simulink model "hybrid1"  (Simulink 8.5)
settings: Solver=ode4  SolverMode=SingleTasking  StartTime=0  StopTime=1369  FixedStep=0.0005  RelTol=1e-3
PreLoadFcn:
  | cd Extensions/Simulink/hybrid1
  | hybrid1_sim_init
  | cd ../../..
undefined symbols (not defined in the file or in its folder): enable_stop, eng_consum_fuel, eng_ctrl_max_trq, eng_idle_spd, eng_map_trq, eng_pwr_max, eng_pwr_opt, eng_spd_opt, ess_cap_scale, ess_fixtemp, ess_init_soc, ess_max_ah_cap, ess_max_volts, ess_min_volts, ess_module_num, ess_res_scale_coef, ess_res_scale_fun, ess_tmp, FR, g_eff_map, g_max_spd, g_max_trq, gc_ki_on, gc_kp_on, I_e, I_g, I_m, I_r, I_R2, m_eff_map, m_map_spd, m_max_trq, m_min_volts, max_gen_spd, min_gen_spd, P_eng_mode, P_ev_mode, regstop_soc, soc_control, target_soc, time_step, tx_pg_r, tx_pg_s, w_engine_on
undefined symbols (not defined in the file): ess_r_chg, ess_r_dis, ess_soc, ess_voc
libraries: Solver_SF x1
(part 1 of 2)
settings Model: Creator=hueipeng  LastModifiedBy=ywata  ExtModeTrigMode=oneshot  ExtModeArmWhenConnect=off
settings DataIOCC: LimitDataPoints=off  SaveOutput=off  SaveTime=off  SignalLoggingName=sigsOut
settings OptimizationCC: BooleanDataType=off  OptimizeBlockIOStorage=off  BufferReuse=off  GlobalBufferReuse=off  ExpressionFolding=off  ExpressionDepthLimit=128  LocalBlockOutputs=off  InitFltsAndDblsToZero=on
settings DebuggingCC: SaveWithParameterizedLinksMsg=none  SignalResolutionControl=TryResolveAllWithWarning  MultiTaskDSMMsg=warning  MultiTaskCondExecSysMsg=none  FcnCallInpInsideContextMsg=EnableAllAsError
settings HardwareCC: TargetUnknown=on
settings GRTTargetCC: TargetFcnLib=ansi_tfl_tmw.mat

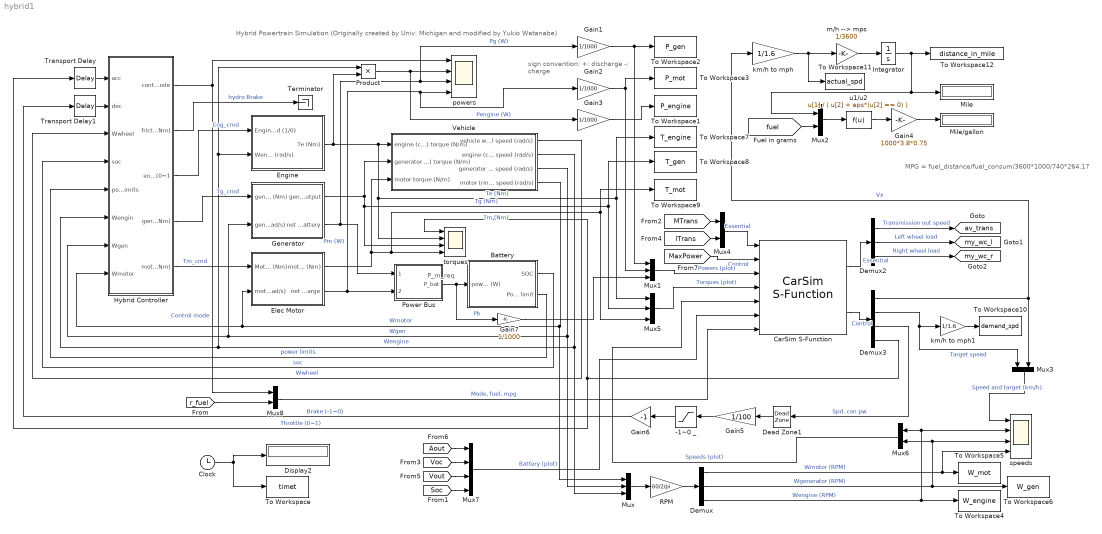
== system hybrid1 ==
  note: Hybrid Powertrain Simulation (Originally created by Univ. Michigan and modified by Yukio Watanabe)
  note: P_m_req
  note: sign convention:
      | +: discharge     -: charge
  note: MPG = fuel_distance/fuel_consum/3600*1000/740*264.17
  -1~0 _ : Saturate  UpperLimit=0  LowerLimit=-1
  Battery : Subsystem
      mask Display: disp('Battery')
  CarSim S-Function : Solver_SF/CarSim S-Function  Priority=1  SIMFILE=simfile.sim
  Clock : Clock
  Dead Zone1 : DeadZone  UpperValue=0  SaturateOnIntegerOverflow=on
  Demux : Demux  Outputs=3
  Demux2 : Demux  Outputs=3
  Demux3 : Demux
  Display2 : Display
  Elec Motor : Subsystem
      mask Display: disp('Electric\nMotor')
  Engine : Subsystem
      mask Display: disp('Engine')
  Gain{1..3,7} (4 alike) : Gain  Gain=1/1000  SaturateOnIntegerOverflow=on  OutDataTypeStr=Inherit: Same as input  ParamDataTypeStr=Inherit: Same as input
  Gain4 : Gain  Gain=1000*3.8*0.75  SaturateOnIntegerOverflow=on  OutDataTypeStr=Inherit: Same as input  ParamDataTypeStr=Inherit: Same as input
  Gain5 : Gain  Gain=1/100  SaturateOnIntegerOverflow=on  OutDataTypeStr=Inherit: Same as input  ParamDataTypeStr=Inherit: Same as input
  Gain6 : Gain  Gain=-1  SaturateOnIntegerOverflow=on  OutDataTypeStr=Inherit: Same as input  ParamDataTypeStr=Inherit: Same as input
  Generator : Subsystem
      mask Display: disp('Generator')
  Hybrid Controller : Subsystem
      mask Display: disp('Hybrid\nController')
  Integrator : Integrator  LowerSaturationLimit=0
  Mile : Display
  Mile/gallon : Display
  Mux : Mux  Inputs=3
  Mux1 : Mux  Inputs=3
  Mux{2..4,6,8} (5 alike) : Mux  Inputs=2
  Mux5 : Mux  Inputs=3
  Mux7 : Mux
  Power Bus : Subsystem
      mask Display: disp('Power\nBus')
  Product : Product  SaturateOnIntegerOverflow=on  OutDataTypeStr=Inherit: Same as first input
  RPM : Gain  Gain=60/2/pi  SaturateOnIntegerOverflow=on  OutDataTypeStr=Inherit: Same as input  ParamDataTypeStr=Inherit: Same as input
  Terminator : Terminator
  To Workspace : ToWorkspace  VariableName=timet  SampleTime=time_step
  To Workspace1 : ToWorkspace  VariableName=P_engine  SampleTime=time_step
  To Workspace10 : ToWorkspace  VariableName=demand_spd  SampleTime=time_step
  To Workspace11 : ToWorkspace  VariableName=actual_spd  SampleTime=time_step
  To Workspace12 : ToWorkspace  VariableName=distance_in_mile  SampleTime=time_step
  To Workspace2 : ToWorkspace  VariableName=P_gen  SampleTime=time_step
  To Workspace3 : ToWorkspace  VariableName=P_mot  SampleTime=time_step
  To Workspace4 : ToWorkspace  VariableName=W_engine  SampleTime=time_step
  To Workspace5 : ToWorkspace  VariableName=W_mot  SampleTime=time_step
  To Workspace6 : ToWorkspace  VariableName=W_gen  SampleTime=time_step
  To Workspace7 : ToWorkspace  VariableName=T_engine  SampleTime=time_step
  To Workspace8 : ToWorkspace  VariableName=T_gen  SampleTime=time_step
  To Workspace9 : ToWorkspace  VariableName=T_mot  SampleTime=time_step
  Transport Delay : TransportDelay  DelayTime=0
  Transport Delay1 : TransportDelay  DelayTime=0
  Vehicle : Subsystem
      mask Display: disp('Planetary Gear Set')
  km/h to mph : Gain  Gain=1/1.6  SaturateOnIntegerOverflow=on  OutDataTypeStr=Inherit: Same as input  ParamDataTypeStr=Inherit: Same as input
  km/h to mph1 : Gain  Gain=1/1.6  SaturateOnIntegerOverflow=on  OutDataTypeStr=Inherit: Same as input  ParamDataTypeStr=Inherit: Same as input
  m/h --> mps : Gain  Gain=1/3600  SaturateOnIntegerOverflow=on  OutDataTypeStr=Inherit: Same as input  ParamDataTypeStr=Inherit: Same as input
  powers : Scope  NumInputPorts=4
      settings: TimeRange=29.9995  YMin=0~0~-20000~-20000  YMax=3~40000~30000~40000  SaveName=ScopeData15
  speeds : Scope  NumInputPorts=4
      settings: TickLabels=on  TimeRange=30  YMin=0~0~-5000~0  YMax=100~4000~10000~6000  SaveName=ScopeData8
  torques : Scope  NumInputPorts=4
      settings: TickLabels=on  TimeRange=29.9995  YMin=0~0~-100~-100  YMax=1~100~50~300  SaveName=ScopeData7
  u1/u2 : Fcn  Expr=u[1] / ( u[2] + eps*(u[2] == 0) )
  tag scope: av_trans=global, my_wc_l=global, my_wc_r=global
  wires:
  Power Bus/1(P_bat) -> Gain7/1, Battery/1(power req'd into bus (W))  "Pb"
  Battery/1(SOC) -> Hybrid Controller/4(soc)  "soc"
  Hybrid Controller/3(engine command (0~1) -> Engine/1(Engine on/off cmd (1/0))  "Eng_cmd"
  Hybrid Controller/4(generator torque command (Nm)) -> Generator/1(generator command Torque (Nm))  "Tg_cmd"
  Hybrid Controller/5(motor torque command (Nm)) -> Elec Motor/1(Motor demand Torque (Nm))  "Tm_cmd"
  Elec Motor/2(net Power >0 discharge  <0 charge) -> Power Bus/2(P_motor), powers/4, Gain2/1  "Pm (W)"
  Generator/2(net Power <0 charge the battery  >0 discharge the battery) -> Power Bus/1(P_generator), powers/3, Gain1/1  "Pg (W)"
  Hybrid Controller/2(friction brake torque (Nm)) -> Terminator/1  "hydro Brake"
  Engine/1(Te (Nm)) -> torques/2, Mux5/1, To Workspace7/1, Vehicle/1(engine (carrier) torque (N/m)), Product/2  "Te (Nm)"
  Vehicle/1(vehicle wheel speed (rad/s)) -> Hybrid Controller/3(Wwheel)  "Wwheel"
  Vehicle/2(engine (carrier) speed (rad/s)) -> Hybrid Controller/6(Wengin), Engine/2(Wengine (rad/s)), Product/1, Mux/3  "Wengine"
  Vehicle/3(generator (sun gear) speed (rad/s)) -> Hybrid Controller/7(Wgen), Generator/2(generator speed (rad/s)), Mux/2  "Wgen"
  Vehicle/4(motor (ring gear) speed (rad/s)) -> Mux/1, Hybrid Controller/8(Wmotor), Elec Motor/2(motor speed (rad/s))  "Wmotor"
  Generator/1(generator torque output) -> torques/3, Mux5/2, To Workspace8/1, Vehicle/2(generator (sun gear) torque (N/m))  "Tg (Nm)"
  Elec Motor/1(motor torque output (Nm)) -> Vehicle/3(motor torque (N/m)), Mux5/3, To Workspace9/1, torques/4  "Tm (Nm)"
  Battery/2(Power limit) -> Hybrid Controller/5(power limits)  "power limits"
  Product/1 -> powers/2, Gain3/1  "Pengine (W)"
  RPM/1 -> Demux/1
  Mux/1 -> RPM/1
  Demux/1 -> speeds/4, To Workspace5/1  "Wmotor (RPM)"
  Demux/2 -> speeds/3, Mux6/2, To Workspace6/1  "Wgenerator (RPM)"
  Demux/3 -> speeds/2, Mux6/1, To Workspace4/1  "Wengine (RPM)"
  Clock/1 -> Display2/1, To Workspace/1
  Gain1/1 -> Mux1/1, To Workspace2/1
  Gain2/1 -> To Workspace3/1, Mux1/2
  Gain3/1 -> To Workspace1/1
  Integrator/1 -> Mux2/1, Mile/1, To Workspace12/1
  [fuel] -> Mux2/2
  u1/u2/1 -> Gain4/1
  Gain4/1 -> Mile/gallon/1
  Mux2/1 -> u1/u2/1
  [MTrans] -> Mux4/1
  Demux2/1 -> [av_trans]  "Transmission out speed"
  Demux2/2 -> [my_wc_l]  "Left wheel load"
  Demux2/3 -> [my_wc_r]  "Right wheel load"
  Demux3/1 -> km/h to mph/1, Mux3/2  "Vx"
  Demux3/4 -> torques/1, Transport Delay/1  "Throttle (0~1)"
  Demux3/2 -> Mux3/1, km/h to mph1/1  "Target speed"
  [ITrans] -> Mux4/2
  [MaxPower] -> CarSim S-Function/2  "Control"
  km/h to mph1/1 -> To Workspace10/1
  Demux3/3 -> Dead Zone1/1  "Spd. con pw"
  Dead Zone1/1 -> Gain5/1
  Gain5/1 -> -1~0 _/1
  -1~0 _/1 -> Gain6/1
  Gain6/1 -> Transport Delay1/1  "Brake (-1~0)"
  m/h --> mps/1 -> Integrator/1
  km/h to mph/1 -> To Workspace11/1, m/h --> mps/1
  Mux3/1 -> speeds/1  "Speed and target (km/h)"
  Transport Delay/1 -> Hybrid Controller/1(acc)
  Transport Delay1/1 -> Hybrid Controller/2(dec)
  Hybrid Controller/1(control mode) -> Mux8/1, powers/1  "Control mode"
  Mux4/1 -> CarSim S-Function/1  "Essential"
  Mux5/1 -> CarSim S-Function/4  "Torques (plot)"
  Mux6/1 -> CarSim S-Function/5  "Speeds (plot)"
  CarSim S-Function/1 -> Demux2/1  "Essential"
  CarSim S-Function/2 -> Demux3/1  "Control"
  Mux1/1 -> CarSim S-Function/3  "Powers (plot)"
  Gain7/1 -> Mux1/3
  [Aout] -> Mux7/1
  [Voc] -> Mux7/2
  [Vout] -> Mux7/3
  [Soc] -> Mux7/4
  Mux7/1 -> CarSim S-Function/6  "Battery (plot)"
  [r_fuel] -> Mux8/2
  Mux8/1 -> CarSim S-Function/7  "Mode, fuel, mpg"

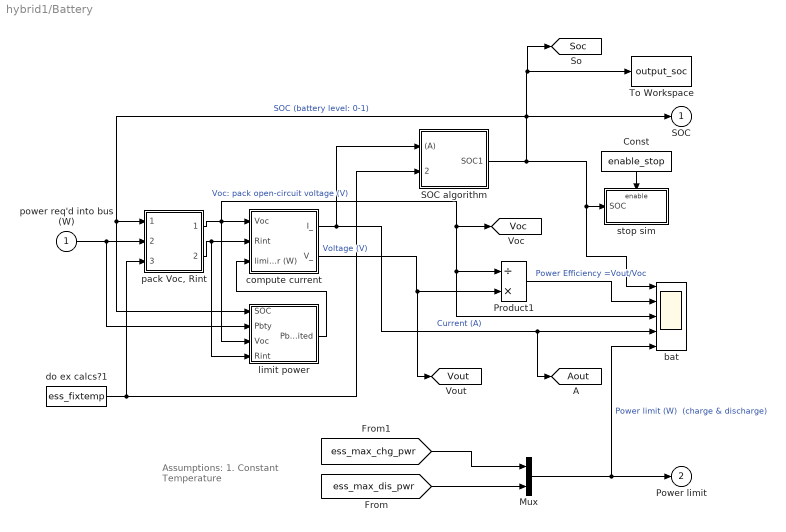
== system hybrid1/Battery ==
  note: Assumptions:
      | 1. Constant Temperature
  power req'd into bus (W) : Inport
  Const : Constant  Value=enable_stop
  Mux : Mux  Inputs=2
  Product1 : Product  Inputs=/*  SaturateOnIntegerOverflow=on  InputSameDT=on  OutDataTypeStr=Inherit: Same as first input
  SOC algorithm : Subsystem  AncestorBlock=|
      | lib_energy_storage/Ess Choices/energy
      | storage <ess>/SOC
      | algorithm
      mask Display: disp('SOC\nalgorithm')
  To Workspace : ToWorkspace  VariableName=output_soc  SampleTime=time_step
  bat : Scope  NumInputPorts=5
      settings: TimeRange=30  YMin=0.5300000000000001~0.6000000000000001~308.8~-50~-50000  YMax=0.6200000000000001~1.2~309.2~100~50000
  compute current : Subsystem  AncestorBlock=|
      | lib_energy_storage/Ess Choices/energy
      | storage <ess>/compute
      | current
      mask Display: disp('Compute\nCurrent')
  do ex calcs?1 : Constant  Value=ess_fixtemp
  limit power : Subsystem  AncestorBlock=lib_energy_storage/Ess Choices/energy storage <ess>/limit power
      mask Display: disp('Limit\nPower')
  "pack Voc, Rint" : Subsystem  AncestorBlock=|
      | lib_energy_storage/Ess Choices/energy
      | storage <ess>/pack
      | Voc, Rint
      mask Display: disp('Pack\nVoc,Rint')
  stop sim : Subsystem  AncestorBlock=lib_energy_storage/Ess Choices/energy storage <ess>/stop sim  TreatAsAtomicUnit=on
  SOC : Outport  InitialOutput=0
  Power limit : Outport  Port=2  InitialOutput=0
  tag scope: Aout=global, Soc=global, Voc=global, Vout=global
  wires:
  limit power/1("Pbty, limited") -> compute current/3(limited output power (W))
  "pack Voc, Rint"/1(pack open- circuit voltage) -> limit power/3(Voc), compute current/1(Voc), Product1/1, bat/3, [Voc]  "Voc: pack open-circuit voltage (V)"
  "pack Voc, Rint"/2(pack resistance) -> compute current/2(Rint), limit power/4(Rint)
  Const/1 -> stop sim/Enable
  SOC algorithm/1(SOC1) -> limit power/1(SOC), "pack Voc, Rint"/1(SOC (prev)), SOC/1, [Soc], To Workspace/1, bat/1, stop sim/1(SOC)  "SOC (battery level: 0-1)"
  compute current/1(I_) -> SOC algorithm/1((A)), [Aout], bat/4  "Current (A)"
  power req'd into bus (W)/1 -> "pack Voc, Rint"/2(req'd battery power (W)), limit power/2(Pbty)
  compute current/2(V_) -> [Vout], Product1/2  "Voltage (V)"
  do ex calcs?1/1 -> "pack Voc, Rint"/3(mod tmp   (C)), SOC algorithm/2(tmp (C))
  Mux/1 -> Power limit/1, bat/5  "Power limit (W)  (charge & discharge)"
  Product1/1 -> bat/2  "Power Efficiency =Vout/Voc"
  [ess_max_dis_pwr] -> Mux/2
  [ess_max_chg_pwr] -> Mux/1

== system hybrid1/Elec Motor ==
  note: disch
  note: charge
  note: discharging
      | power
  Motor demand Torque (Nm) : Inport
  motor speed (rad/s) : Inport  Port=2
  Abs : Abs  SaturateOnIntegerOverflow=on
  Efficiency Look-Up Table (2-D) : Lookup2D  RowIndex=m_map_spd  ColumnIndex=m_map_trq  Table=m_eff_map  SaturateOnIntegerOverflow=on  InputSameDT=on
  First-order lag : TransferFcn  Denominator=[0.05 1]
  MinMax : MinMax  Inputs=2  SaturateOnIntegerOverflow=on  InputSameDT=on
  Power out  is > 0 or < 0 ? : Switch  SaturateOnIntegerOverflow=on  InputSameDT=on
  Product1 : Product  Inputs=*/  SaturateOnIntegerOverflow=on  InputSameDT=on  OutDataTypeStr=Inherit: Same as first input
  Sign : Signum
  charging power : Product  SaturateOnIntegerOverflow=on  InputSameDT=on  OutDataTypeStr=Inherit: Same as first input
  max torque : Lookup  InputValues=m_map_spd  Table=m_max_trq  SaturateOnIntegerOverflow=on
  motoring or braking torque2 : Product  SaturateOnIntegerOverflow=on  InputSameDT=on  OutDataTypeStr=Inherit: Same as first input
  power1 : Product  SaturateOnIntegerOverflow=on  InputSameDT=on  OutDataTypeStr=Inherit: Same as first input
  motor torque output (Nm) : Outport  InitialOutput=0
  net Power >0 discharge  <0 charge : Outport  Port=2  InitialOutput=0
  wires:
  charging power/1 -> Power out  is > 0 or < 0 ?/3
  Product1/1 -> Power out  is > 0 or < 0 ?/1
  Power out  is > 0 or < 0 ?/1 -> net Power >0 discharge  <0 charge/1  "power to/from battery (W)"
  motor speed (rad/s)/1 -> Efficiency Look-Up Table (2-D)/1, motoring or braking torque2/1, max torque/1  "motor speed"
  Motor demand Torque (Nm)/1 -> Abs/1, Sign/1
  power1/1 -> First-order lag/1  "torque"
  Efficiency Look-Up Table (2-D)/1 -> Product1/2, charging power/2
  motoring or braking torque2/1 -> Product1/1, charging power/1, Power out  is > 0 or < 0 ?/2
  Abs/1 -> MinMax/2
  max torque/1 -> MinMax/1
  MinMax/1 -> power1/1
  Sign/1 -> power1/2
  First-order lag/1 -> Efficiency Look-Up Table (2-D)/2, motoring or braking torque2/2, motor torque output (Nm)/1

== system hybrid1/Engine ==
  note: MPG = fuel_distance/fuel_consum/3600*1000/740*264.17
  Engine on/off cmd (1/0) : Inport
  Wengine (rad/s) : Inport  Port=2
  Gain : Gain  Gain=1/1000
  Integrator : Integrator  UpperSaturationLimit=20.5  LowerSaturationLimit=0
  Scope : Scope
      settings: SaveName=ScopeData13
  To Workspace : ToWorkspace  VariableName=fuel_consum_in_g  SampleTime=time_step
  "We, Te to fuel" : Lookup2D  RowIndex=eng_consum_spd  ColumnIndex=eng_consum_trq  Table=eng_consum_fuel  SaturateOnIntegerOverflow=on  InputSameDT=on
  "fuel, speed to T" : Lookup2D  RowIndex=eng_map_spd  ColumnIndex=eng_map_fuel  Table=eng_map_trq  SaturateOnIntegerOverflow=on  InputSameDT=on
  Te (Nm) : Outport
  tag scope: fuel=global, r_fuel=global
  wires:
  Engine on/off cmd (1/0)/1 -> Scope/1, "fuel, speed to T"/2
  Wengine (rad/s)/1 -> "fuel, speed to T"/1, "We, Te to fuel"/1
  "fuel, speed to T"/1 -> Te (Nm)/1, "We, Te to fuel"/2
  "We, Te to fuel"/1 -> Gain/1, Integrator/1
  Integrator/1 -> To Workspace/1, [fuel]
  Gain/1 -> [r_fuel]

== system hybrid1/Generator ==
  note: disch
  note: charge
  note: discharging
      | power
  generator command Torque (Nm) : Inport
  generator speed (rad/s) : Inport  Port=2
  Abs : Abs  SaturateOnIntegerOverflow=on
  Efficiency Look-Up Table (2-D) : Lookup2D  RowIndex=g_map_spd  ColumnIndex=g_map_trq  Table=g_eff_map  SaturateOnIntegerOverflow=on  InputSameDT=on
  First-order lag : TransferFcn  Denominator=[0.05 1]
  MinMax : MinMax  Inputs=2  SaturateOnIntegerOverflow=on  InputSameDT=on
  Power out  is > 0 or < 0 ? : Switch  SaturateOnIntegerOverflow=on  InputSameDT=on
  Product1 : Product  Inputs=*/  SaturateOnIntegerOverflow=on  InputSameDT=on  OutDataTypeStr=Inherit: Same as first input
  Sign : Signum
  charging power : Product  SaturateOnIntegerOverflow=on  InputSameDT=on  OutDataTypeStr=Inherit: Same as first input
  max torque : Lookup  InputValues=g_max_spd  Table=g_max_trq  SaturateOnIntegerOverflow=on
  motoring or braking torque2 : Product  SaturateOnIntegerOverflow=on  InputSameDT=on  OutDataTypeStr=Inherit: Same as first input
  power1 : Product  SaturateOnIntegerOverflow=on  InputSameDT=on  OutDataTypeStr=Inherit: Same as first input
  generator torque output : Outport  InitialOutput=0
  net Power <0 charge the battery  >0 discharge the battery : Outport  Port=2  InitialOutput=0
  wires:
  charging power/1 -> Power out  is > 0 or < 0 ?/3
  Product1/1 -> Power out  is > 0 or < 0 ?/1
  Power out  is > 0 or < 0 ?/1 -> net Power <0 charge the battery  >0 discharge the battery/1  "power to/from battery (W)"
  generator speed (rad/s)/1 -> Efficiency Look-Up Table (2-D)/1, motoring or braking torque2/1, max torque/1  "generator speed"
  generator command Torque (Nm)/1 -> Abs/1, Sign/1
  power1/1 -> First-order lag/1  "torque"
  Efficiency Look-Up Table (2-D)/1 -> Product1/2, charging power/2
  motoring or braking torque2/1 -> Product1/1, charging power/1, Power out  is > 0 or < 0 ?/2
  Abs/1 -> MinMax/2
  max torque/1 -> MinMax/1
  MinMax/1 -> power1/1
  Sign/1 -> power1/2
  First-order lag/1 -> generator torque output/1, Efficiency Look-Up Table (2-D)/2, motoring or braking torque2/2

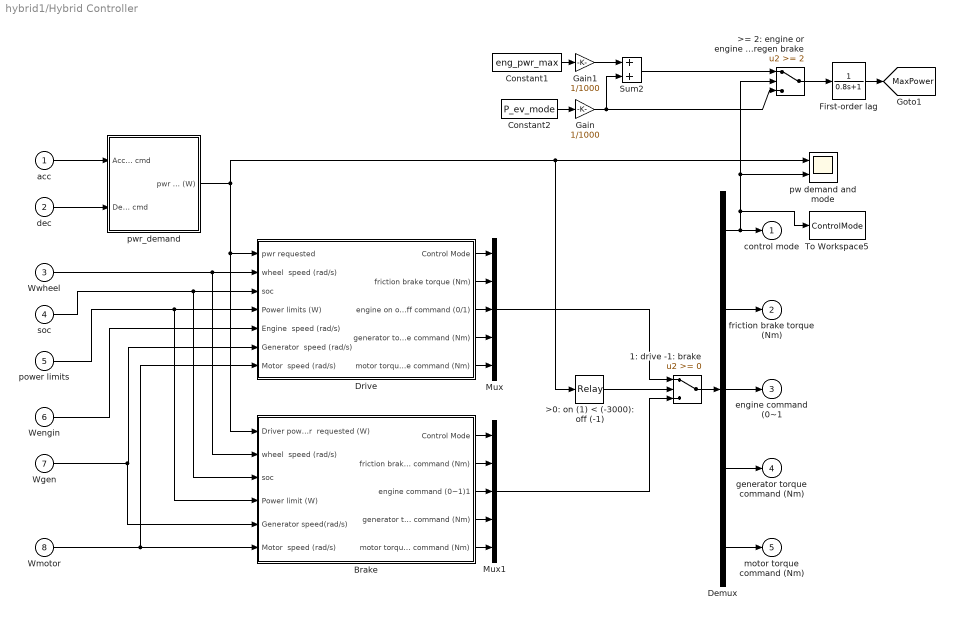
== system hybrid1/Hybrid Controller ==
  acc : Inport
  dec : Inport  Port=2
  Wwheel : Inport  Port=3
  soc : Inport  Port=4
  power limits : Inport  Port=5
  Wengin : Inport  Port=6
  Wgen : Inport  Port=7
  Wmotor : Inport  Port=8
  1: drive -1: brake : Switch  SaturateOnIntegerOverflow=on
  >0: on (1) < (-3000): off (-1) : Relay  OnSwitchValue=0  OffSwitchValue=-3000  OffOutputValue=-1
  >= 2: engine or engine + motor; < 2: motor only or regen brake : Switch  Threshold=2  SaturateOnIntegerOverflow=on
  Brake : Subsystem  AncestorBlock=|
      | lib_controls/<vc> prius/Coordinated
      |  Controller/max engine
      | efficiency point
      mask Display: disp('Braking\nControl')
  Constant1 : Constant  Value=eng_pwr_max
  Constant2 : Constant  Value=P_ev_mode
  Demux : Demux  Outputs=5
  Drive : Subsystem  AncestorBlock=|
      | lib_controls/<vc> prius/Coordinated
      |  Controller/max engine
      | efficiency point
      mask Display: disp('Driving\nControl')
  First-order lag : TransferFcn  Denominator=[0.8 1]
  Gain : Gain  Gain=1/1000
  Gain1 : Gain  Gain=1/1000
  Mux : Mux  Inputs=5
  Mux1 : Mux  Inputs=5
  Sum2 : Sum  SaturateOnIntegerOverflow=on  InputSameDT=on  OutDataTypeStr=Inherit: Same as first input
  To Workspace5 : ToWorkspace  VariableName=ControlMode  SampleTime=time_step
  pw demand and mode : Scope  NumInputPorts=2
      settings: TimeRange=30  YMin=-10000~0  YMax=60000~3  SaveName=ScopeData17
  pwr_demand : Subsystem
      mask Display: disp('Power\nDemand')
  control mode : Outport
  friction brake torque (Nm) : Outport  Port=2
  engine command (0~1 : Outport  Port=3
  generator torque command (Nm) : Outport  Port=4
  motor torque command (Nm) : Outport  Port=5
  tag scope: MaxPower=global
  wires:
  pwr_demand/1(pwr dmd (W)) -> Drive/1(pwr requested), Brake/1(Driver power  requested (W)), >0: on (1) < (-3000): off (-1)/1, pw demand and mode/1
  acc/1 -> pwr_demand/1(Accel cmd)
  Drive/1(Control Mode) -> Mux/1
  Drive/2(friction brake torque (Nm)) -> Mux/2
  Drive/3(engine on off command (0/1)) -> Mux/3
  Drive/4(generator torque command (Nm)) -> Mux/4
  Drive/5(motor torque command (Nm)) -> Mux/5
  Brake/1(Control Mode) -> Mux1/1
  Brake/2(friction brake torque command (Nm)) -> Mux1/2
  Brake/3(engine command (0~1)1) -> Mux1/3
  Brake/4(generator torque command (Nm)) -> Mux1/4
  Brake/5(motor torque command (Nm)) -> Mux1/5
  Mux/1 -> 1: drive -1: brake/1
  Mux1/1 -> 1: drive -1: brake/3
  1: drive -1: brake/1 -> Demux/1
  Demux/1 -> >= 2: engine or engine + motor; < 2: motor only or regen brake/2, pw demand and mode/2, To Workspace5/1, control mode/1
  Demux/2 -> friction brake torque (Nm)/1
  Wwheel/1 -> Drive/2(wheel  speed (rad/s)), Brake/2(wheel  speed (rad/s))
  soc/1 -> Drive/3(soc), Brake/3(soc)
  power limits/1 -> Drive/4(Power limits (W)), Brake/4(Power limit (W))
  Wengin/1 -> Drive/5(Engine  speed (rad/s))
  Wgen/1 -> Brake/5(Generator speed(rad/s)), Drive/6(Generator  speed (rad/s))
  Wmotor/1 -> Brake/6(Motor  speed (rad/s)), Drive/7(Motor  speed (rad/s))
  dec/1 -> pwr_demand/2(Decel cmd)
  >0: on (1) < (-3000): off (-1)/1 -> 1: drive -1: brake/2
  Constant1/1 -> Gain1/1
  Constant2/1 -> Gain/1
  >= 2: engine or engine + motor; < 2: motor only or regen brake/1 -> First-order lag/1
  Gain/1 -> Sum2/2, >= 2: engine or engine + motor; < 2: motor only or regen brake/3
  Gain1/1 -> Sum2/1
  Sum2/1 -> >= 2: engine or engine + motor; < 2: motor only or regen brake/1
  First-order lag/1 -> [MaxPower]
  Demux/3 -> engine command (0~1/1
  Demux/4 -> generator torque command (Nm)/1
  Demux/5 -> motor torque command (Nm)/1

== system hybrid1/Power Bus ==
  P_generator : Inport
  P_motor : Inport  Port=2
  Gain3 : Gain  Gain=1/1000  SaturateOnIntegerOverflow=on  OutDataTypeStr=Inherit: Same as input  ParamDataTypeStr=Inherit: Same as input
  Sum : Sum  SaturateOnIntegerOverflow=on  InputSameDT=on  OutDataTypeStr=Inherit: Same as first input
  To Workspace : ToWorkspace  VariableName=P_batt  SampleTime=time_step
  P_bat : Outport  InitialOutput=0
  wires:
  P_generator/1 -> Sum/1
  P_motor/1 -> Sum/2
  Sum/1 -> P_bat/1, Gain3/1  "Batt"
  Gain3/1 -> To Workspace/1

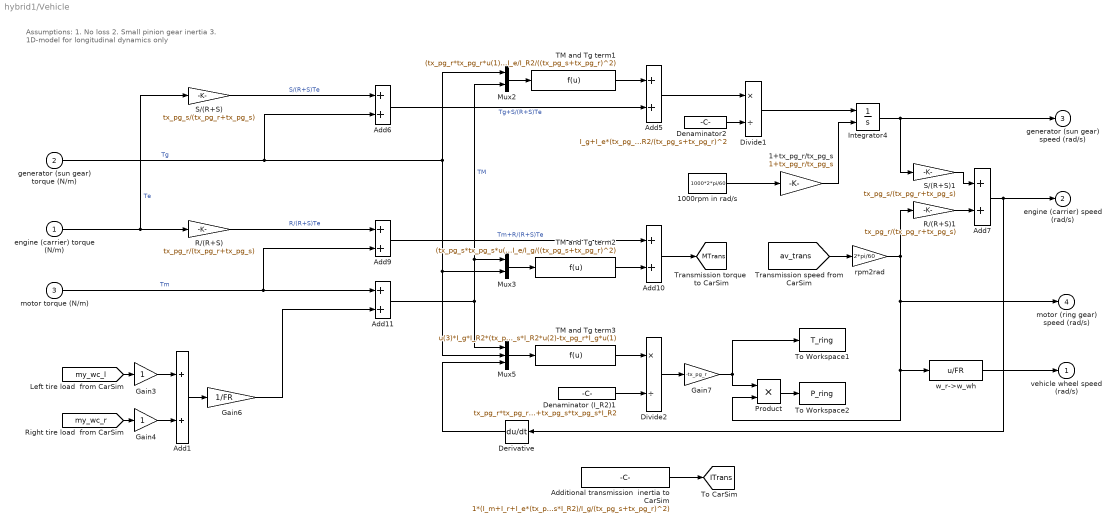
== system hybrid1/Vehicle ==
  note: Assumptions:
      | 1. No loss
      | 2. Small pinion gear inertia
      | 3. 1D-model for longitudinal dynamics only
  engine (carrier) torque (N/m) : Inport
  generator (sun gear) torque (N/m) : Inport  Port=2
  motor torque (N/m) : Inport  Port=3
  1+tx_pg_r/tx_pg_s : Gain  Gain=1+tx_pg_r/tx_pg_s  SaturateOnIntegerOverflow=on  OutDataTypeStr=Inherit: Same as input  ParamDataTypeStr=Inherit: Same as input
  1000rpm in rad/s : Constant  Value=1000*2*pi/60
  Add{1,5..7,9..11} (7 alike) : Sum
  Additional transmission  inertia to CarSim : Constant  Value=1*(I_m+I_r+I_e*(tx_pg_r*tx_pg_r*I_g+tx_pg_s*tx_pg_s*I_R2)/I_g/(tx_pg_s+tx_pg_r)^2)
  Denaminator (I_R2)1 : Constant  Value=tx_pg_r*tx_pg_r*I_g+tx_pg_s*tx_pg_s*I_R2
  Denaminator2 : Constant  Value=I_g+I_e*(tx_pg_r*tx_pg_r*I_g+tx_pg_s*tx_pg_s*I_R2)/I_R2/(tx_pg_s+tx_pg_r)^2
  Derivative : Derivative
  Divide1 : Product  Inputs=*/
  Divide2 : Product  Inputs=*/
  Gain3 : Gain
  Gain4 : Gain
  Gain6 : Gain  Gain=1/FR  SaturateOnIntegerOverflow=on  OutDataTypeStr=Inherit: Same as input  ParamDataTypeStr=Inherit: Same as input
  Gain7 : Gain  Gain=-tx_pg_r  SaturateOnIntegerOverflow=on  OutDataTypeStr=Inherit: Same as input  ParamDataTypeStr=Inherit: Same as input
  Integrator4 : Integrator  InitialConditionSource=external  LimitOutput=on
  Mux2 : Mux  Inputs=2
  Mux3 : Mux  Inputs=2
  Mux5 : Mux  Inputs=3
  Product : Product  SaturateOnIntegerOverflow=on  InputSameDT=on  OutDataTypeStr=Inherit: Same as first input
  R/(R+S) : Gain  Gain=tx_pg_r/(tx_pg_r+tx_pg_s)  SaturateOnIntegerOverflow=on  OutDataTypeStr=Inherit: Same as input  ParamDataTypeStr=Inherit: Same as input
  R/(R+S)1 : Gain  Gain=tx_pg_r/(tx_pg_r+tx_pg_s)  SaturateOnIntegerOverflow=on  OutDataTypeStr=Inherit: Same as input  ParamDataTypeStr=Inherit: Same as input
  S/(R+S) : Gain  Gain=tx_pg_s/(tx_pg_r+tx_pg_s)  SaturateOnIntegerOverflow=on  OutDataTypeStr=Inherit: Same as input  ParamDataTypeStr=Inherit: Same as input
  S/(R+S)1 : Gain  Gain=tx_pg_s/(tx_pg_r+tx_pg_s)  SaturateOnIntegerOverflow=on  OutDataTypeStr=Inherit: Same as input  ParamDataTypeStr=Inherit: Same as input
  TM and Tg term1 : Fcn  Expr=(tx_pg_r*tx_pg_r*u(1)-tx_pg_r*tx_pg_s*u(2)) *I_e/I_R2/((tx_pg_s+tx_pg_r)^2)
  TM and Tg term2 : Fcn  Expr=(tx_pg_s*tx_pg_s*u(1)-tx_pg_r*tx_pg_s*u(2)) *I_e/I_g/((tx_pg_s+tx_pg_r)^2)
  TM and Tg term3 : Fcn  Expr=u(3)*I_g*I_R2*(tx_pg_r+tx_pg_s)-tx_pg_s*I_R2*u(2)-tx_pg_r*I_g*u(1)
  To Workspace1 : ToWorkspace  VariableName=T_ring  SampleTime=time_step
  To Workspace2 : ToWorkspace  VariableName=P_ring  SampleTime=time_step
  rpm2rad : Gain  Gain=2*pi/60  SaturateOnIntegerOverflow=on  OutDataTypeStr=Inherit: Same as input  ParamDataTypeStr=Inherit: Same as input
  w_r->w_wh : Fcn  Expr=u/FR
  vehicle wheel speed (rad/s) : Outport
  engine (carrier) speed (rad/s) : Outport  Port=2
  generator (sun gear) speed (rad/s) : Outport  Port=3
  motor (ring gear) speed (rad/s) : Outport  Port=4
  tag scope: ITrans=global, MTrans=global
  wires:
  w_r->w_wh/1 -> vehicle wheel speed (rad/s)/1
  Add7/1 -> engine (carrier) speed (rad/s)/1, Derivative/1
  rpm2rad/1 -> Product/2, w_r->w_wh/1, motor (ring gear) speed (rad/s)/1, R/(R+S)1/1
  Integrator4/1 -> generator (sun gear) speed (rad/s)/1, S/(R+S)1/1
  Product/1 -> To Workspace2/1
  Gain7/1 -> To Workspace1/1, Product/1
  Divide2/1 -> Gain7/1
  Denaminator (I_R2)1/1 -> Divide2/2
  TM and Tg term3/1 -> Divide2/1
  Derivative/1 -> Mux5/3
  Mux5/1 -> TM and Tg term3/1
  Add11/1 -> Mux3/1, Mux2/2, Mux5/1  "TM"
  Mux3/1 -> TM and Tg term2/1
  TM and Tg term2/1 -> Add10/2
  Additional transmission  inertia to CarSim/1 -> [ITrans]
  Add10/1 -> [MTrans]
  Add9/1 -> Add10/1  "Tm+R/(R+S)Te"
  Gain6/1 -> Add11/2
  1+tx_pg_r/tx_pg_s/1 -> Integrator4/2
  R/(R+S)1/1 -> Add7/2
  S/(R+S)1/1 -> Add7/1
  1000rpm in rad/s/1 -> 1+tx_pg_r/tx_pg_s/1
  Denaminator2/1 -> Divide1/2
  Mux2/1 -> TM and Tg term1/1
  Divide1/1 -> Integrator4/1
  Add5/1 -> Divide1/1
  TM and Tg term1/1 -> Add5/1
  Add6/1 -> Add5/2  "Tg+S/(R+S)Te"
  S/(R+S)/1 -> Add6/1  "S/(R+S)Te"
  Gain4/1 -> Add1/2
  Gain3/1 -> Add1/1
  Add1/1 -> Gain6/1
  [my_wc_l] -> Gain3/1
  [my_wc_r] -> Gain4/1
  [av_trans] -> rpm2rad/1
  R/(R+S)/1 -> Add9/1  "R/(R+S)Te"
  engine (carrier) torque (N/m)/1 -> S/(R+S)/1, R/(R+S)/1  "Te"
  generator (sun gear) torque (N/m)/1 -> Add6/2, Mux5/2, Mux3/2, Mux2/1  "Tg"
  motor torque (N/m)/1 -> Add9/2, Add11/1  "Tm"

== system hybrid1/Battery/SOC algorithm ==
  note: SOC=(Max Ah capacity-Ah used)/Max Ah capacity
  (A) : Inport
  tmp (C) : Inport  Port=2
  (sec->hrs) : Gain  Gain=1/3600  SaturateOnIntegerOverflow=on  OutDataTypeStr=Inherit: Same as input  ParamDataTypeStr=Inherit: Same as input
  0 <= SOC <= 1 : Saturate  UpperLimit=1  LowerLimit=0
  A-h remaining : Sum  Inputs=-+  SaturateOnIntegerOverflow=on  InputSameDT=on  OutDataTypeStr=Inherit: Same as first input
  Ah used : Integrator  InitialConditionSource=external  InitialCondition=(1-ess_init_soc)*ess_max_ah_cap
  Fcn : Fcn  Expr=1/u
  Fcn1 : Fcn  Expr=(1-ess_init_soc)*u
  SOC : Product  SaturateOnIntegerOverflow=on  InputSameDT=on  OutDataTypeStr=Inherit: Same as first input
  max cap : Lookup  InputValues=ess_tmp  Table=ess_max_ah_cap*ess_cap_scale  SaturateOnIntegerOverflow=on
  SOC1 : Outport  InitialOutput=0
  wires:
  (A)/1 -> (sec->hrs)/1
  (sec->hrs)/1 -> Ah used/1
  Ah used/1 -> A-h remaining/1
  Fcn/1 -> SOC/2
  SOC/1 -> 0 <= SOC <= 1/1
  A-h remaining/1 -> SOC/1
  0 <= SOC <= 1/1 -> SOC1/1
  tmp (C)/1 -> max cap/1
  max cap/1 -> A-h remaining/2, Fcn/1, Fcn1/1
  Fcn1/1 -> Ah used/2

== system hybrid1/Battery/compute current ==
  Voc : Inport
  Rint : Inport  Port=2
  limited output power (W) : Inport  Port=3
  Ibty=(Voc-(Voc^2-4RPbty)^.5)        ----------------------------- (2*R) : Fcn  Expr=(u[2]-(u[2]^2-4*u[1]*u[3])^.5)/(2*u[3])
  Memory : Memory
  Mux3 : Mux  Inputs=3
  Mux4 : Mux  Inputs=3
  Mux5 : Mux  Inputs=3
  Pch_max=Imax*Vmax : Product  SaturateOnIntegerOverflow=on  InputSameDT=on  OutDataTypeStr=Inherit: Same as first input
  Voc-I*R : Fcn  Expr=u[2]-u[1]*u[3]
  ess max voltage*#batts : Constant  Value=ess_max_volts*ess_module_num
  iabs min=(Voc-Vmax)/R : Fcn  Expr=(u(1)-u(2))/u(3)
  limit current based on  max voltage during charge : Switch  Threshold=eps  SaturateOnIntegerOverflow=on  InputSameDT=on
  min charge current not exceeded : RelationalOperator  Operator=>  InputSameDT=on
  I_ : Outport  InitialOutput=0
  V_ : Outport  Port=2  InitialOutput=0
  tag scope: ess_max_chg_pwr=global
  wires:
  limited output power (W)/1 -> Mux4/1
  Voc/1 -> Mux4/2, Mux3/2, Mux5/1
  Rint/1 -> Mux4/3, Mux3/3, Mux5/3
  Ibty=(Voc-(Voc^2-4RPbty)^.5)        ----------------------------- (2*R)/1 -> min charge current not exceeded/1, limit current based on  max voltage during charge/1
  iabs min=(Voc-Vmax)/R/1 -> min charge current not exceeded/2, limit current based on  max voltage during charge/3, Pch_max=Imax*Vmax/1
  limit current based on  max voltage during charge/1 -> Mux3/1, I_/1
  min charge current not exceeded/1 -> limit current based on  max voltage during charge/2
  Mux3/1 -> Voc-I*R/1
  Voc-I*R/1 -> V_/1
  Mux4/1 -> Ibty=(Voc-(Voc^2-4RPbty)^.5)        ----------------------------- (2*R)/1
  Mux5/1 -> iabs min=(Voc-Vmax)/R/1
  ess max voltage*#batts/1 -> Mux5/2, Pch_max=Imax*Vmax/2
  Pch_max=Imax*Vmax/1 -> Memory/1
  Memory/1 -> [ess_max_chg_pwr]

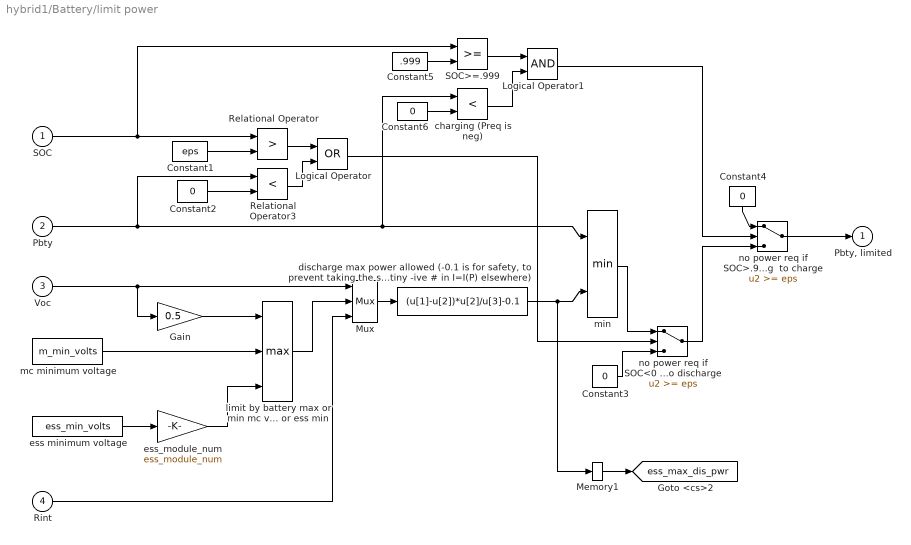
== system hybrid1/Battery/limit power ==
  SOC : Inport
  Pbty : Inport  Port=2
  Voc : Inport  Port=3
  Rint : Inport  Port=4
  Constant1 : Constant  Value=eps
  Constant{2..4,6} (4 alike) : Constant  Value=0
  Constant5 : Constant  Value=.999
  Gain : Gain  Gain=0.5  SaturateOnIntegerOverflow=on  OutDataTypeStr=Inherit: Same as input  ParamDataTypeStr=Inherit: Same as input
  Logical Operator : Logic  Operator=OR
  Logical Operator1 : Logic
  Memory1 : Memory
  Mux : Mux  Inputs=3
  Relational Operator : RelationalOperator  Operator=>  InputSameDT=on
  Relational Operator3 : RelationalOperator  Operator=<  InputSameDT=on
  SOC>=.999 : RelationalOperator  InputSameDT=on
  charging (Preq is neg) : RelationalOperator  Operator=<  InputSameDT=on
  "discharge max power allowed (-0.1 is for safety, to prevent taking the square of a tiny -ive # in I=I(P) elsewhere)" : Fcn  Expr=(u[1]-u[2])*u[2]/u[3]-0.1
  ess minimum voltage : Constant  Value=ess_min_volts
  ess_module_num : Gain  Gain=ess_module_num  SaturateOnIntegerOverflow=on  OutDataTypeStr=Inherit: Same as input  ParamDataTypeStr=Inherit: Same as input
  limit by battery max or min mc voltage or ess min : MinMax  Function=max  Inputs=3  SaturateOnIntegerOverflow=on  InputSameDT=on
  mc minimum voltage : Constant  Value=m_min_volts
  min : MinMax  Inputs=2  SaturateOnIntegerOverflow=on  InputSameDT=on
  no power req if SOC<0 and trying  to discharge : Switch  Threshold=eps  SaturateOnIntegerOverflow=on  InputSameDT=on
  no power req if SOC>.999 and trying  to charge : Switch  Threshold=eps  SaturateOnIntegerOverflow=on  InputSameDT=on
  "Pbty, limited" : Outport  InitialOutput=0
  tag scope: ess_max_dis_pwr=global
  wires:
  Constant1/1 -> Relational Operator/2
  Relational Operator/1 -> Logical Operator/1
  Pbty/1 -> Relational Operator3/1, charging (Preq is neg)/1, min/1
  Constant2/1 -> Relational Operator3/2
  Relational Operator3/1 -> Logical Operator/2
  Constant3/1 -> no power req if SOC<0 and trying  to discharge/3
  Logical Operator/1 -> no power req if SOC<0 and trying  to discharge/2
  Voc/1 -> Mux/1, Gain/1
  min/1 -> no power req if SOC<0 and trying  to discharge/1
  Mux/1 -> "discharge max power allowed (-0.1 is for safety, to prevent taking the square of a tiny -ive # in I=I(P) elsewhere)"/1
  limit by battery max or min mc voltage or ess min/1 -> Mux/2
  "discharge max power allowed (-0.1 is for safety, to prevent taking the square of a tiny -ive # in I=I(P) elsewhere)"/1 -> min/2, Memory1/1
  mc minimum voltage/1 -> limit by battery max or min mc voltage or ess min/2
  Rint/1 -> Mux/3
  Gain/1 -> limit by battery max or min mc voltage or ess min/1
  ess minimum voltage/1 -> ess_module_num/1
  ess_module_num/1 -> limit by battery max or min mc voltage or ess min/3
  SOC/1 -> Relational Operator/1, SOC>=.999/1
  SOC>=.999/1 -> Logical Operator1/1
  Constant6/1 -> charging (Preq is neg)/2
  charging (Preq is neg)/1 -> Logical Operator1/2
  Constant5/1 -> SOC>=.999/2
  Constant4/1 -> no power req if SOC>.999 and trying  to charge/1
  no power req if SOC<0 and trying  to discharge/1 -> no power req if SOC>.999 and trying  to charge/3
  no power req if SOC>.999 and trying  to charge/1 -> "Pbty, limited"/1
  Logical Operator1/1 -> no power req if SOC>.999 and trying  to charge/2
  Memory1/1 -> [ess_max_dis_pwr]

== system hybrid1/Battery/pack Voc, Rint ==
  SOC (prev) : Inport
  req'd battery power (W) : Inport  Port=2
  mod tmp   (C) : Inport  Port=3
  #bty : Constant  Value=ess_module_num
  Product : Product  SaturateOnIntegerOverflow=on  InputSameDT=on  OutDataTypeStr=Inherit: Same as first input
  Rchg (ohms) : Subsystem  mask(2-D Table Lookup){xindex=ess_tmp, yindex=ess_soc, table=ess_r_chg}
      mask prompts: xindex "X Index"; yindex "Y Index"
      mask help:
      | Two Dimensional Table Lookup
      | The first input corresponds to X Index and the second input corresponds to the Y Index
      mask init:
      | sftab2chk(xindex,yindex,table);
      mask Help: This block returns a linearly interpolated intersection from the table using the X index (which corresponds to the rows of the table) and the Y index (which corresponds to the columns of the table).  Extrapolation is used.
      mask Display: plot(-10,-10,110,110,[90,50,10],[90,40,30],[90,50,10],[50,26,20],[90,50,10],[22,13,10])
  Rdis (ohms) : Subsystem  mask(2-D Table Lookup){xindex=ess_tmp, yindex=ess_soc, table=ess_r_dis}
      mask prompts: xindex "X Index"; yindex "Y Index"
      mask help:
      | Two Dimensional Table Lookup
      | The first input corresponds to X Index and the second input corresponds to the Y Index
      mask init:
      | sftab2chk(xindex,yindex,table);
      mask Help: This block returns a linearly interpolated intersection from the table using the X index (which corresponds to the rows of the table) and the Y index (which corresponds to the columns of the table).  Extrapolation is used.
      mask Display: plot(-10,-10,110,110,[90,50,10],[90,40,30],[90,50,10],[50,26,20],[90,50,10],[22,13,10])
  Switch : Switch  SaturateOnIntegerOverflow=on  InputSameDT=on
  VOC (V) : Subsystem  mask(2-D Table Lookup){xindex=ess_tmp, yindex=ess_soc, table=ess_voc}
      mask prompts: xindex "X Index"; yindex "Y Index"
      mask help:
      | Two Dimensional Table Lookup
      | The first input corresponds to X Index and the second input corresponds to the Y Index
      mask init:
      | sftab2chk(xindex,yindex,table);
      mask Help: This block returns a linearly interpolated intersection from the table using the X index (which corresponds to the rows of the table) and the Y index (which corresponds to the columns of the table).  Extrapolation is used.
      mask Display: plot(-10,-10,110,110,[90,50,10],[90,40,30],[90,50,10],[50,26,20],[90,50,10],[22,13,10])
  resistance scale fun : Gain  Gain=ess_res_scale_fun(ess_res_scale_coef,ess_module_num,ess_cap_scale)  SaturateOnIntegerOverflow=on  OutDataTypeStr=Inherit: Same as input  ParamDataTypeStr=Inherit: Same as input
  resistance scale fun1 : Gain  Gain=ess_res_scale_fun(ess_res_scale_coef,ess_module_num,ess_cap_scale)  SaturateOnIntegerOverflow=on  OutDataTypeStr=Inherit: Same as input  ParamDataTypeStr=Inherit: Same as input
  pack open- circuit voltage : Outport  InitialOutput=0
  pack resistance : Outport  Port=2  InitialOutput=0
  wires:
  resistance scale fun1/1 -> Switch/3
  Rchg (ohms)/1(table out) -> resistance scale fun1/1
  resistance scale fun/1 -> Switch/1
  Rdis (ohms)/1(table out) -> resistance scale fun/1
  Switch/1 -> pack resistance/1
  #bty/1 -> Product/2
  Product/1 -> pack open- circuit voltage/1
  VOC (V)/1(table out) -> Product/1
  req'd battery power (W)/1 -> Switch/2
  SOC (prev)/1 -> VOC (V)/2(y0), Rdis (ohms)/2(y0), Rchg (ohms)/2(y0)
  mod tmp   (C)/1 -> VOC (V)/1(x0), Rdis (ohms)/1(x0), Rchg (ohms)/1(x0)

== system hybrid1/Battery/stop sim ==
  SOC : Inport
  Enable : EnablePort
  Const : Constant  Value=.001
  Relational Operator : RelationalOperator  Operator=<  InputSameDT=on
  Stop Simulation : Stop
  wires:
  Const/1 -> Relational Operator/2
  SOC/1 -> Relational Operator/1
  Relational Operator/1 -> Stop Simulation/1

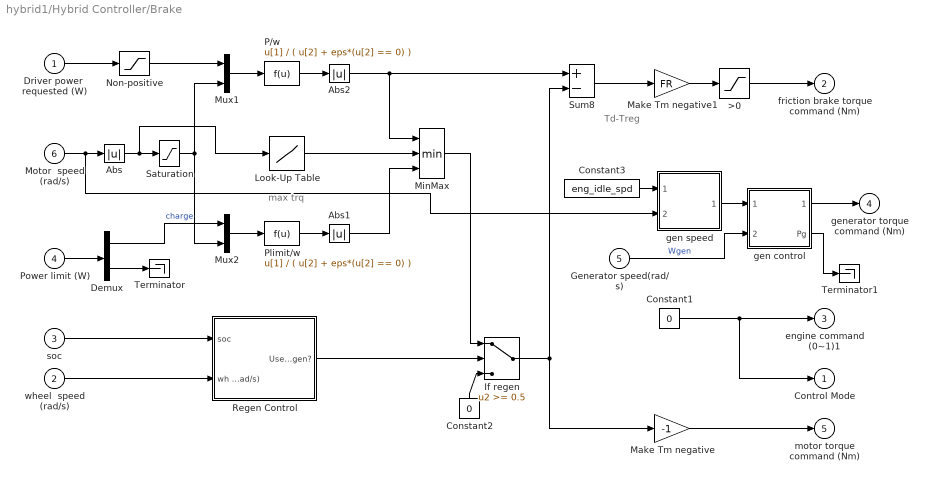
== system hybrid1/Hybrid Controller/Brake ==
  note: max trq
  note: Td-Treg
  Driver power  requested (W) : Inport
  wheel  speed (rad/s) : Inport  Port=2
  soc : Inport  Port=3
  Power limit (W) : Inport  Port=4
  Generator speed(rad/s) : Inport  Port=5
  Motor  speed (rad/s) : Inport  Port=6
  >0 : Saturate  UpperLimit=10000  LowerLimit=0
  Abs : Abs  SaturateOnIntegerOverflow=on
  Abs1 : Abs  SaturateOnIntegerOverflow=on
  Abs2 : Abs  SaturateOnIntegerOverflow=on
  Constant1 : Constant  Value=0
  Constant2 : Constant  Value=0
  Constant3 : Constant  Value=eng_idle_spd
  Demux : Demux  Outputs=2
  If regen : Switch  Threshold=0.5  SaturateOnIntegerOverflow=on  InputSameDT=on
  Look-Up Table : Lookup  InputValues=m_map_spd  Table=m_max_trq  SaturateOnIntegerOverflow=on
  Make Tm negative : Gain  Gain=-1  SaturateOnIntegerOverflow=on  OutDataTypeStr=Inherit: Same as input  ParamDataTypeStr=Inherit: Same as input
  Make Tm negative1 : Gain  Gain=FR  SaturateOnIntegerOverflow=on  OutDataTypeStr=Inherit: Same as input  ParamDataTypeStr=Inherit: Same as input
  MinMax : MinMax  Inputs=3  SaturateOnIntegerOverflow=on  InputSameDT=on
  Mux1 : Mux  Inputs=2
  Mux2 : Mux  Inputs=2
  Non-positive : Saturate  UpperLimit=0  LowerLimit=-inf
  P/w : Fcn  Expr=u[1] / ( u[2] + eps*(u[2] == 0) )
  Plimit/w : Fcn  Expr=u[1] / ( u[2] + eps*(u[2] == 0) )
  Regen Control : Subsystem
      mask Display: disp('Regen\nControl')
  Saturation : Saturate  UpperLimit=inf  LowerLimit=10
  Sum8 : Sum  Inputs=+-  SaturateOnIntegerOverflow=on  InputSameDT=on  OutDataTypeStr=Inherit: Same as first input
  Terminator : Terminator
  Terminator1 : Terminator
  gen control : Subsystem  AncestorBlock=|
      | lib_controls/<vc> prius/Coordinated
      |  Controller/max engine
      | efficiency point
      mask Display: disp('M/G1\nControl')
  gen speed : Subsystem  AncestorBlock=|
      | lib_controls/<vc> prius/Coordinated
      |  Controller/max engine
      | efficiency point
      mask Display: disp('Target\nM/G1\nSpeed')
  Control Mode : Outport
  friction brake torque command (Nm) : Outport  Port=2
  engine command (0~1)1 : Outport  Port=3
  generator torque command (Nm) : Outport  Port=4
  motor torque command (Nm) : Outport  Port=5
  wires:
  Mux1/1 -> P/w/1
  Non-positive/1 -> Mux1/1
  P/w/1 -> Abs2/1
  Constant2/1 -> If regen/3
  MinMax/1 -> If regen/1
  Demux/1 -> Mux2/1  "charge"
  Power limit (W)/1 -> Demux/1
  If regen/1 -> Make Tm negative/1, Sum8/2
  Abs2/1 -> MinMax/1, Sum8/1
  Motor  speed (rad/s)/1 -> gen speed/2(Ring Gear/Motor current speed (rad/s)), Abs/1
  Abs/1 -> Look-Up Table/1, Saturation/1
  Make Tm negative1/1 -> >0/1
  Sum8/1 -> Make Tm negative1/1
  Look-Up Table/1 -> MinMax/2
  wheel  speed (rad/s)/1 -> Regen Control/2(wh spd (rad/s))
  Plimit/w/1 -> Abs1/1
  Abs1/1 -> MinMax/3
  Driver power  requested (W)/1 -> Non-positive/1
  soc/1 -> Regen Control/1(soc)
  >0/1 -> friction brake torque command (Nm)/1
  Make Tm negative/1 -> motor torque command (Nm)/1
  Constant1/1 -> Control Mode/1, engine command (0~1)1/1
  Mux2/1 -> Plimit/w/1
  Demux/2 -> Terminator/1
  Regen Control/1("Use regen? ") -> If regen/2
  Saturation/1 -> Mux1/2, Mux2/2
  gen speed/1(Reference generator speed (rad/s)) -> gen control/1(Reference speed (rad/s))
  Constant3/1 -> gen speed/1(Target engine speed (rad/s))
  Generator speed(rad/s)/1 -> gen control/2(Generator current  speed (rad/s))  "Wgen"
  gen control/1(generator torque command (Nm)) -> generator torque command (Nm)/1
  gen control/2(Pg) -> Terminator1/1

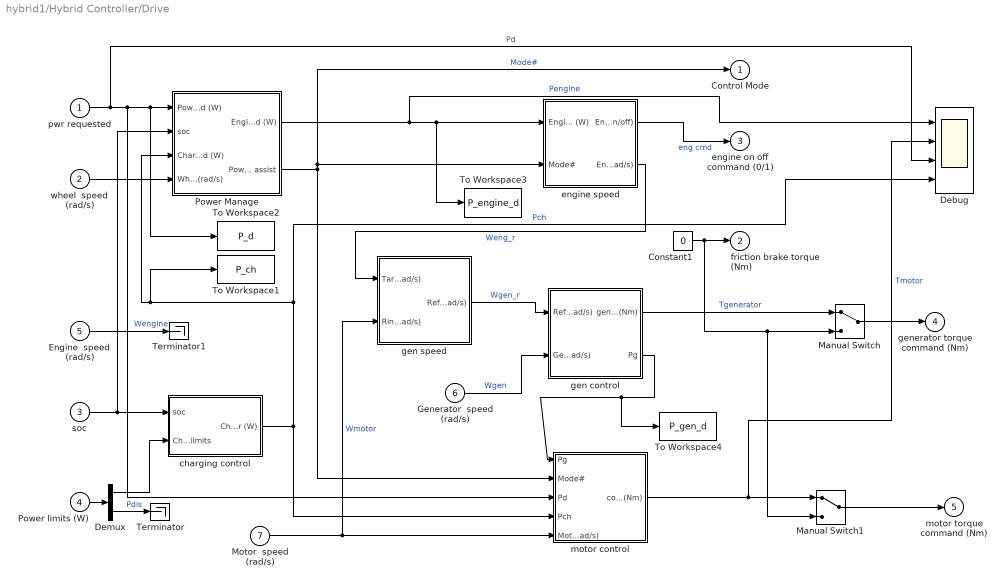
== system hybrid1/Hybrid Controller/Drive ==
  pwr requested : Inport
  wheel  speed (rad/s) : Inport  Port=2
  soc : Inport  Port=3
  Power limits (W) : Inport  Port=4
  Engine  speed (rad/s) : Inport  Port=5
  Generator  speed (rad/s) : Inport  Port=6
  Motor  speed (rad/s) : Inport  Port=7
  Constant1 : Constant  Value=0
  Debug : Scope  NumInputPorts=4
      settings: TimeRange=30  YMin=0~0~-20000~0  YMax=40000~400~60000~10000  SaveName=ScopeData18
  Demux : Demux  Outputs=2
  Manual Switch : ManualSwitch
  Manual Switch1 : ManualSwitch
  Power Manage : Subsystem
      mask Display: disp('Power\nManagement\nControl')
  Terminator : Terminator
  Terminator1 : Terminator
  To Workspace1 : ToWorkspace  VariableName=P_ch  SampleTime=time_step
  To Workspace2 : ToWorkspace  VariableName=P_d  SampleTime=time_step
  To Workspace3 : ToWorkspace  VariableName=P_engine_d  SampleTime=time_step
  To Workspace4 : ToWorkspace  VariableName=P_gen_d  SampleTime=time_step
  charging control : Subsystem  AncestorBlock=|
      | lib_controls/<vc> prius/Coordinated
      |  Controller/max engine
      | efficiency point
      mask Display: disp('Battery\ncharge\nDemand')
  engine speed : Subsystem
      mask Display: disp('Engine\nOptimal\nControl')
  gen control : Subsystem  AncestorBlock=|
      | lib_controls/<vc> prius/Coordinated
      |  Controller/max engine
      | efficiency point
      mask Display: disp('M/G1\nControl')
  gen speed : Subsystem  AncestorBlock=|
      | lib_controls/<vc> prius/Coordinated
      |  Controller/max engine
      | efficiency point
      mask Display: disp('Target\nM/G1\nSpeed')
  motor control : Subsystem  AncestorBlock=|
      | lib_controls/<vc> prius/Coordinated
      |  Controller/max engine
      | efficiency point
      mask Display: disp('M/G2\nControl')
  Control Mode : Outport
  friction brake torque (Nm) : Outport  Port=2
  engine on off command (0/1) : Outport  Port=3
  generator torque command (Nm) : Outport  Port=4
  motor torque command (Nm) : Outport  Port=5
  wires:
  Constant1/1 -> Manual Switch1/2, Manual Switch/2, friction brake torque (Nm)/1
  gen control/1(generator torque command (Nm)) -> Manual Switch/1  "Tgenerator"
  motor control/1(command motor torque (Nm)) -> Manual Switch1/1, Debug/2  "Tmotor"
  gen speed/1(Reference generator speed (rad/s)) -> gen control/1(Reference speed (rad/s))  "Wgen_r"
  Generator  speed (rad/s)/1 -> gen control/2(Generator current  speed (rad/s))  "Wgen"
  soc/1 -> Power Manage/2(soc), charging control/1(soc)
  Power Manage/1(Engine Power demand (W)) -> engine speed/1(Engine Power Demand (W)), To Workspace3/1, Debug/1  "Pengine"
  charging control/1(Charging Power (W)) -> To Workspace1/1, Power Manage/3(Charging power demand (W)), Debug/4, motor control/4(Pch)  "Pch"
  Motor  speed (rad/s)/1 -> gen speed/2(Ring Gear/Motor current speed (rad/s)), motor control/5(Motor  speed (rad/s))  "Wmotor"
  pwr requested/1 -> motor control/3(Pd), Power Manage/1(Power demand (W)), To Workspace2/1, Debug/3  "Pd"
  engine speed/1(Engine Cmd (on/off)) -> engine on off command (0/1)/1  "eng cmd"
  engine speed/2(Engine operating speed (rad/s)) -> gen speed/1(Target engine speed (rad/s))  "Weng_r"
  Power Manage/2(Power Mode 1: Motor only 2: Engine only 3: Power assist) -> engine speed/2(Mode#), Control Mode/1, motor control/2(Mode#)  "Mode#"
  Engine  speed (rad/s)/1 -> Terminator1/1  "Wengine"
  Power limits (W)/1 -> Demux/1
  Demux/1 -> charging control/2(Charging power limits)
  Demux/2 -> Terminator/1  "Pdis"
  gen control/2(Pg) -> To Workspace4/1, motor control/1(Pg)
  Manual Switch/1 -> generator torque command (Nm)/1
  Manual Switch1/1 -> motor torque command (Nm)/1
  wheel  speed (rad/s)/1 -> Power Manage/4(Wheel Speed (rad/s))

== system hybrid1/Hybrid Controller/pwr_demand ==
  note: max_brake_power
  note: >0:acc; <0:brake
  Accel cmd : Inport
  Decel cmd : Inport  Port=2
  Constant : Constant  Value=55000
  Max braking torqu : Gain  Gain=80000  SaturateOnIntegerOverflow=on  OutDataTypeStr=Inherit: Same as input  ParamDataTypeStr=Inherit: Same as input
  Product : Product  SaturateOnIntegerOverflow=on  InputSameDT=on  OutDataTypeStr=Inherit: Same as first input
  Sum6 : Sum  Inputs=|+-  SaturateOnIntegerOverflow=on  InputSameDT=on  OutDataTypeStr=Inherit: Same as first input
  pwr dmd (W) : Outport
  wires:
  Decel cmd/1 -> Max braking torqu/1
  Accel cmd/1 -> Product/2
  Product/1 -> Sum6/1
  Max braking torqu/1 -> Sum6/2
  Constant/1 -> Product/1  "Max Driving Power (Pengine+Pbattery)"
  Sum6/1 -> pwr dmd (W)/1

== system hybrid1/Battery/pack Voc, Rint/Rchg (ohms) ==
  x0 : Inport
  y0 : Inport  Port=2
  Mux : Mux  Inputs=2
  S-function : S-Function  FunctionName=sftable2  Parameters=xindex, yindex, table
  table out : Outport  InitialOutput=0
  wires:
  y0/1 -> Mux/2
  S-function/1 -> table out/1
  x0/1 -> Mux/1
  Mux/1 -> S-function/1

== system hybrid1/Battery/pack Voc, Rint/Rdis (ohms) ==
  x0 : Inport
  y0 : Inport  Port=2
  Mux : Mux  Inputs=2
  S-function : S-Function  FunctionName=sftable2  Parameters=xindex, yindex, table
  table out : Outport  InitialOutput=0
  wires:
  y0/1 -> Mux/2
  S-function/1 -> table out/1
  x0/1 -> Mux/1
  Mux/1 -> S-function/1

== system hybrid1/Battery/pack Voc, Rint/VOC (V) ==
  x0 : Inport
  y0 : Inport  Port=2
  Mux : Mux  Inputs=2
  S-function : S-Function  FunctionName=sftable2  Parameters=xindex, yindex, table
  table out : Outport  InitialOutput=0
  wires:
  y0/1 -> Mux/2
  S-function/1 -> table out/1
  x0/1 -> Mux/1
  Mux/1 -> S-function/1

== system hybrid1/Hybrid Controller/Brake/Regen Control ==
  soc : Inport
  wh spd (rad/s) : Inport  Port=2
  Logical Operator : Logic  Inputs=3
  regen swith on : Constant
  soc condition : Relay  OnSwitchValue=regstop_soc*1.1  OffSwitchValue=regstop_soc  OnOutputValue=0  OffOutputValue=1
  wheel spd>= 0.4 : Relay  OnSwitchValue=0.4  OffSwitchValue=0.2
  "Use regen? " : Outport
  wires:
  wh spd (rad/s)/1 -> wheel spd>= 0.4/1
  soc/1 -> soc condition/1
  wheel spd>= 0.4/1 -> Logical Operator/1
  Logical Operator/1 -> "Use regen? "/1
  soc condition/1 -> Logical Operator/2
  regen swith on/1 -> Logical Operator/3

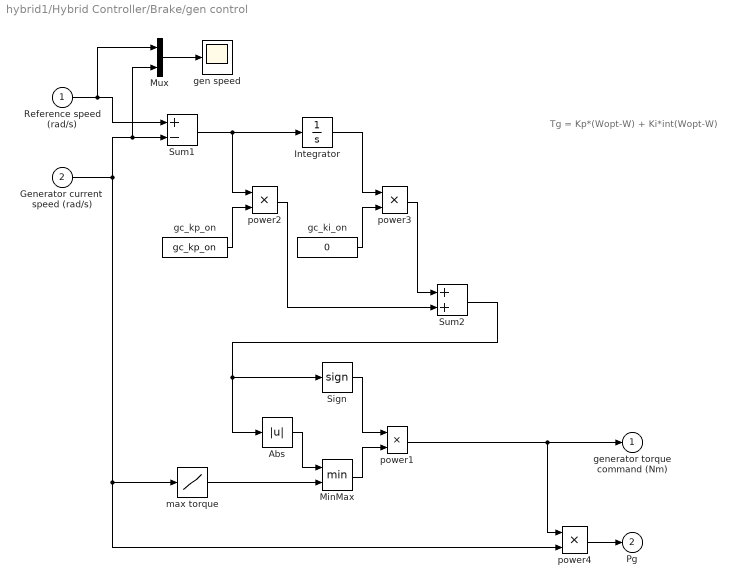
== system hybrid1/Hybrid Controller/Brake/gen control ==
  note: Tg = Kp*(Wopt-W) + Ki*int(Wopt-W)
  Reference speed (rad/s) : Inport
  Generator current  speed (rad/s) : Inport  Port=2
  Abs : Abs  SaturateOnIntegerOverflow=on
  Integrator : Integrator
  MinMax : MinMax  Inputs=2  SaturateOnIntegerOverflow=on  InputSameDT=on
  Mux : Mux  Inputs=2
  Sign : Signum
  Sum1 : Sum  Inputs=+-  SaturateOnIntegerOverflow=on  InputSameDT=on  OutDataTypeStr=Inherit: Same as first input
  Sum2 : Sum  SaturateOnIntegerOverflow=on  InputSameDT=on  OutDataTypeStr=Inherit: Same as first input
  gc_ki_on : Constant  Value=0
  gc_kp_on : Constant  Value=gc_kp_on
  gen speed : Scope
      settings: YMin=50  YMax=900  SaveName=ScopeData14
  max torque : Lookup  InputValues=g_max_spd  Table=g_max_trq  SaturateOnIntegerOverflow=on
  power{1..4} (4 alike) : Product  SaturateOnIntegerOverflow=on  InputSameDT=on  OutDataTypeStr=Inherit: Same as first input
  generator torque command (Nm) : Outport
  Pg : Outport  Port=2
  wires:
  Abs/1 -> MinMax/1
  max torque/1 -> MinMax/2
  Sign/1 -> power1/1
  MinMax/1 -> power1/2
  Reference speed (rad/s)/1 -> Sum1/1, Mux/1
  Generator current  speed (rad/s)/1 -> Sum1/2, Mux/2, max torque/1, power4/2
  Sum1/1 -> power2/1, Integrator/1
  gc_kp_on/1 -> power2/2
  gc_ki_on/1 -> power3/2
  Integrator/1 -> power3/1
  power3/1 -> Sum2/1
  power2/1 -> Sum2/2
  Sum2/1 -> Sign/1, Abs/1
  Mux/1 -> gen speed/1
  power1/1 -> generator torque command (Nm)/1, power4/1
  power4/1 -> Pg/1

== system hybrid1/Hybrid Controller/Brake/gen speed ==
  Target engine speed (rad/s) : Inport
  Ring Gear/Motor current speed (rad/s) : Inport  Port=2
  1+tx_pg_r/tx_pg_s : Gain  Gain=1+tx_pg_r/tx_pg_s  SaturateOnIntegerOverflow=on  OutDataTypeStr=Inherit: Same as input  ParamDataTypeStr=Inherit: Same as input
  Saturation min_gen,max_gen : Saturate  UpperLimit=max_gen_spd*0.9  LowerLimit=min_gen_spd*0.9
  Sum1 : Sum  Inputs=+-  SaturateOnIntegerOverflow=on  InputSameDT=on  OutDataTypeStr=Inherit: Same as first input
  tx_pg_r/tx_pg_s : Gain  Gain=tx_pg_r/tx_pg_s  SaturateOnIntegerOverflow=on  OutDataTypeStr=Inherit: Same as input  ParamDataTypeStr=Inherit: Same as input
  Reference generator speed (rad/s) : Outport
  wires:
  Saturation min_gen,max_gen/1 -> Reference generator speed (rad/s)/1
  tx_pg_r/tx_pg_s/1 -> Sum1/2
  1+tx_pg_r/tx_pg_s/1 -> Sum1/1
  Target engine speed (rad/s)/1 -> 1+tx_pg_r/tx_pg_s/1
  Sum1/1 -> Saturation min_gen,max_gen/1
  Ring Gear/Motor current speed (rad/s)/1 -> tx_pg_r/tx_pg_s/1
